simulink model "EstimadorFriccion"  (R2015a)
settings: Solver=ode45  StartTime=0.0  StopTime=40  FixedStep=0.0001  MinStep=0.001  RelTol=1e-3
libraries: simulink x3, cstblocks x1
settings Model: Creator=Usuario  LastModifiedBy=Usuario

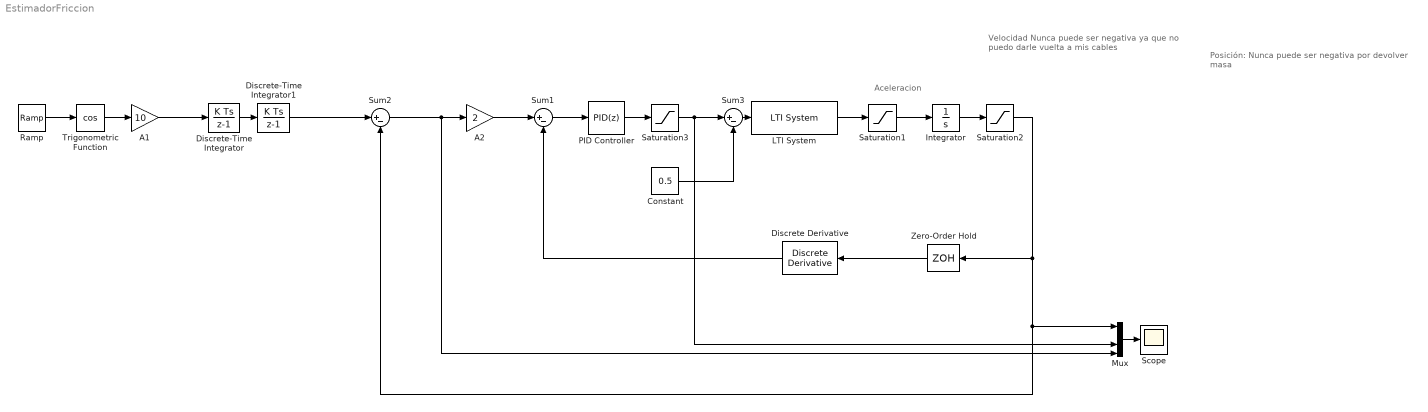
== system EstimadorFriccion ==
  note: Posición:
      | Nunca puede ser negativa por devolver masa
  note: Velocidad
      | Nunca puede ser negativa ya que no puedo
      | darle vuelta a mis cables
  note: Aceleracion
  A1 : Gain  Gain=10
  A2 : Gain  Gain=2
  Constant : Constant  Value=0.5
  Discrete Derivative : simulink/Discrete/Discrete Derivative  gainval=1.0  ICPrevScaledInput=0.0  InputProcessing=Inherited  OutMin=[]  OutMax=[]  OutDataType=fixdt(1, 16)  OutScaling=2^-10  DoSatur=off
  Discrete-Time Integrator : DiscreteIntegrator  InitialConditionSetting=State (most efficient)  SampleTime=0.05
  Discrete-Time Integrator1 : DiscreteIntegrator  InitialConditionSetting=State (most efficient)  SampleTime=0.05
  Integrator : Integrator
  LTI System : cstblocks/LTI System  sys=Vs  IC=[]
  Mux : Mux
  PID Controller : simulink/Continuous/PID Controller  Controller=PID  TimeDomain=Discrete-time  SampleTime=0.05  IntegratorMethod=Backward Euler  FilterMethod=Backward Euler  Form=Parallel  UseFilter=on  ControllerParametersSource=internal  P=1  I=0.1  D=0.4  N=100  InitialConditionSource=internal  InitialConditionForIntegrator=0  InitialConditionForFilter=0  ExternalReset=none  LimitOutput=off  UpperSaturationLimit=inf  LowerSaturationLimit=-inf  LinearizeAsGain=on  AntiWindupMode=none  Kb=1  TrackingMode=off  Kt=1  PParamMin=[]  PParamMax=[]  IParamMin=[]  IParamMax=[]  DParamMin=[]  DParamMax=[]  NParamMin=[]  NParamMax=[]  KbParamMin=[]  KbParamMax=[]  KtParamMin=[]  KtParamMax=[]  POutMin=[]  POutMax=[]  IOutMin=[]  IOutMax=[]  DOutMin=[]  DOutMax=[]  NOutMin=[]  NOutMax=[]  KbOutMin=[]  KbOutMax=[]  KtOutMin=[]  KtOutMax=[]  IntegratorOutMin=[]  IntegratorOutMax=[]  FilterOutMin=[]  FilterOutMax=[]  SumOutMin=[]  SumOutMax=[]  SumI1OutMin=[]  SumI1OutMax=[]  SumI2OutMin=[]  SumI2OutMax=[]  SumI3OutMin=[]  SumI3OutMax=[]  SumDOutMin=[]  SumDOutMax=[]  SaturationOutMin=[]  SaturationOutMax=[]  IntegratorContinuousStateAttributes=''  IntegratorStateMustResolveToSignalObject=off  IntegratorRTWStateStorageClass=Auto  FilterContinuousStateAttributes=''  FilterStateMustResolveToSignalObject=off  FilterRTWStateStorageClass=Auto  DifferentiatorICPrevScaledInput=0  DifferentiatorOutMin=[]  DifferentiatorOutMax=[]
  Ramp : simulink/Sources/Ramp  slope=0.1  start=0  X0=0
  Saturation1 : Saturate  UpperLimit=100000  LowerLimit=0
  Saturation2 : Saturate  UpperLimit=100000  LowerLimit=0
  Saturation3 : Saturate  UpperLimit=1  LowerLimit=0
  Scope : Scope
      settings: TimeRange=10  YMin=-3.480473123841992e-52  YMax=0.0002877639694426701  MaxDataPoints=50000
  Sum1 : Sum  Inputs=|+-
  Sum2 : Sum  Inputs=|+-
  Sum3 : Sum  Inputs=|+-
  Trigonometric Function : Trigonometry  Operator=cos
  Zero-Order Hold : ZeroOrderHold  SampleTime=0.05
  wires:
  Trigonometric Function/1 -> A1/1
  Mux/1 -> Scope/1
  Ramp/1 -> Trigonometric Function/1
  A1/1 -> Discrete-Time Integrator/1
  Sum2/1 -> A2/1, Mux/4
  Discrete-Time Integrator1/1 -> Sum2/1
  Discrete-Time Integrator/1 -> Discrete-Time Integrator1/1
  A2/1 -> Sum1/1
  LTI System/1 -> Saturation1/1
  Saturation1/1 -> Integrator/1
  Integrator/1 -> Saturation2/1
  Sum1/1 -> PID Controller/1
  Saturation2/1 -> Zero-Order Hold/1, Mux/1, Sum2/2
  PID Controller/1 -> Saturation3/1
  Saturation3/1 -> Mux/3, Sum3/1
  Sum3/1 -> LTI System/1
  Constant/1 -> Sum3/2
  Zero-Order Hold/1 -> Discrete Derivative/1
  Discrete Derivative/1 -> Sum1/2
